simulink model "logdemo"  (Simulink 6.0)
settings: Solver=VariableStepDiscrete  SolverMode=SingleTasking  StartTime=0.0  StopTime=100  RelTol=1e-3  AbsTol=1e-6
libraries: simulink_extras x4
settings Model: CovMetricSettings=d  Creator=The MathWorks Inc.  LastModifiedBy=batserve  ExtModeTrigMode=oneshot  ExtModeArmWhenConnect=off  ExtModeAutoUpdateStatusClock=off
settings DataIOCC: ExternalInput=[]  InitialState=[]  LimitDataPoints=off  SaveOutput=off  SaveTime=off
settings OptimizationCC: BlockReduction=off
settings DebuggingCC: CheckExecutionContextPreStartOutputMsg=on  CheckExecutionContextRuntimeOutputMsg=on  SolverPrmCheckMsg=none  IntegerOverflowMsg=none  UnconnectedOutputMsg=none
settings HardwareCC: TargetUnknown=on

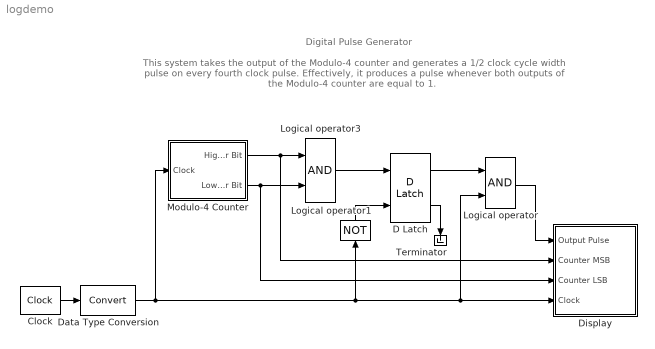
== system logdemo ==
  note: This system takes the output of the Modulo-4 counter and
      | generates a 1/2 clock cycle width pulse on every fourth clock pulse.
      | Effectively, it produces a pulse whenever both outputs of the
      | Modulo-4 counter are equal to 1.
  note: Digital Pulse Generator
  Clock : simulink_extras/Flip Flops/Clock  MaskParam1=1
  D Latch : simulink_extras/Flip Flops/D Latch
  Data Type Conversion : DataTypeConversion  OutDataTypeMode=boolean  SaturateOnIntegerOverflow=on  RndMeth=Zero
  Display : Subsystem  PropExecContextAcrossSSBoundary=on
  Logical operator : Logic
  Logical operator1 : Logic  Orientation=up  Operator=NOT  Inputs=1
  Logical operator3 : Logic
  Modulo-4 Counter : Subsystem  PropExecContextAcrossSSBoundary=on
  Terminator : Terminator
      settings: Orientation=down
  wires:
  Logical operator3/1 -> D Latch/1
  Logical operator1/1 -> D Latch/2
  D Latch/1 -> Logical operator/1
  Logical operator/1 -> Display/1(Output Pulse)
  Modulo-4 Counter/2(Low-Order Bit) -> Logical operator3/2, Display/3(Counter LSB)
  Clock/1 -> Data Type Conversion/1
  Modulo-4 Counter/1(High-Order Bit) -> Logical operator3/1, Display/2(Counter MSB)
  D Latch/2 -> Terminator/1
  Data Type Conversion/1 -> Logical operator1/1, Display/4(Clock), Logical operator/2, Modulo-4 Counter/1(Clock)

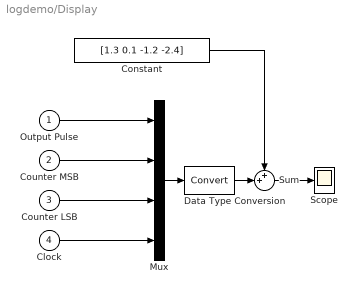
== system logdemo/Display ==
  Output Pulse : Inport  Port=1  LatchInput=off
  Counter MSB : Inport  Port=2  LatchInput=off
  Counter LSB : Inport  Port=3  LatchInput=off
  Clock : Inport  Port=4  LatchInput=off
  Constant : Constant  Value=[1.3 0.1 -1.2 -2.4]
  Data Type Conversion : DataTypeConversion  OutDataTypeMode=double  SaturateOnIntegerOverflow=on  RndMeth=Zero
  Mux : Mux
  Scope : Scope
      settings: TickLabels=on  TimeRange=100  YMin=-3  YMax=3  DataFormat=Array
  Sum : Sum  Inputs=++|  SaturateOnIntegerOverflow=on  InputSameDT=on
  wires:
  Sum/1 -> Scope/1
  Counter MSB/1 -> Mux/2
  Counter LSB/1 -> Mux/3
  Clock/1 -> Mux/4
  Constant/1 -> Sum/1
  Mux/1 -> Data Type Conversion/1
  Output Pulse/1 -> Mux/1
  Data Type Conversion/1 -> Sum/2

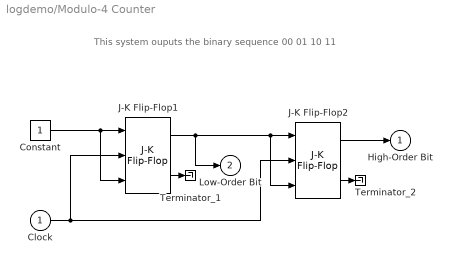
== system logdemo/Modulo-4 Counter ==
  note: This system ouputs the binary sequence
      | 00 01 10 11
  Clock : Inport  Port=1  LatchInput=off
  Constant : Constant  OutDataTypeMode=boolean
  J-K Flip-Flop1 : simulink_extras/Flip Flops/J-K Flip-Flop  initial_condition=0
  J-K Flip-Flop2 : simulink_extras/Flip Flops/J-K Flip-Flop  initial_condition=0
  Terminator_1 : Terminator
  Terminator_2 : Terminator
  High-Order Bit : Outport  InitialOutput=0
  Low-Order Bit : Outport  Port=2  InitialOutput=0
  wires:
  J-K Flip-Flop2/2 -> Terminator_2/1
  J-K Flip-Flop1/2 -> Terminator_1/1
  J-K Flip-Flop1/1 -> Low-Order Bit/1, J-K Flip-Flop2/3, J-K Flip-Flop2/1
  Constant/1 -> J-K Flip-Flop1/1, J-K Flip-Flop1/3
  Clock/1 -> J-K Flip-Flop1/2, J-K Flip-Flop2/2
  J-K Flip-Flop2/1 -> High-Order Bit/1
